simulink library "motor_lib"  (Simulink 7.8)
settings: Solver=ode45  StartTime=0.0  StopTime=10.0  RelTol=1e-3
libraries: powerlib x8
settings Model: Creator=re25624  LastModifiedBy=ma25949

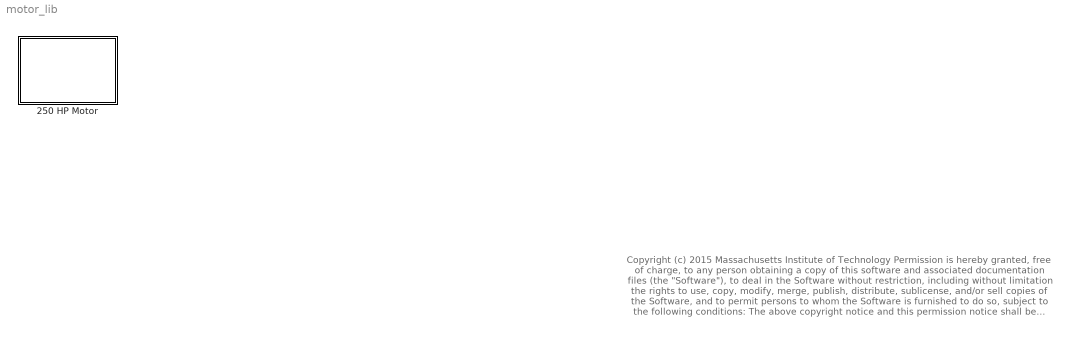
== system motor_lib ==
  note: Copyright (c) 2015 Massachusetts Institute of Technology
      | Permission is hereby granted, free of charge, to any person obtaining a copy of this software and associated documentation files (the "Software"), to deal in the Software without restriction, including without limitation the rights to use, copy, modify, merge, publish, distribute, sublicense, and/or sell copies of the Software, and to permit persons to whom the Software is furnished to do so, subject to the following conditions:
      |
      | The above copyright notice and this permission notice shall be included in all copies or substantial portions of the Software.
      |
      | THE SOFTWARE IS PROVIDED "AS IS", WITHOUT WARRANTY OF ANY KIND, EXPRESS OR IMPLIED, INCLUDING BUT NOT LIMITED TO THE WARRANTIES OF MERCHANTABILITY, FITNESS FOR A PARTICULAR PURPOSE AND NONINFRINGEMENT. IN NO EVENT SHALL THE AUTHORS OR COPYRIGHT HOLDERS BE LIABLE FOR ANY CLAIM,
      | DAMAGES OR OTHER LIABILITY, WHETHER IN AN ACTION OF CONTRACT, TORT OR OTHERWISE, ARISING FROM, OUT OF OR IN CONNECTION WITH THE SOFTWARE OR THE USE OR OTHER DEALINGS IN THE SOFTWARE.
  250 HP Motor : Subsystem  mask(SimPowersystems 250 HP custom motor){H=0.03}
      mask prompts: H "Inertia [Sec]"
      mask help:
      | This motor was built using parameters from the EPTM motor models.
      |
      | To keep this model stable, the inertia must be suffiently high. Otherwise, after the initial step the solution will be invalid and noisy. Also note that adding input filters appears to cause the solution to ring.
      |
      | When connecting this motor to an inductive load (such as a transformer), a capacitive load is necessary for the solvers to work properly.
      mask Display:
      | disp('250 HP\nmotor')
      | port_label('LConn', 1, 'A')
      | port_label('LConn', 2, 'B')
      | port_label('LConn', 3, 'C')

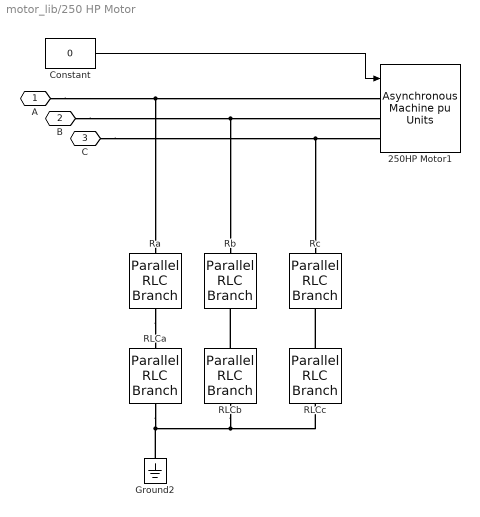
== system motor_lib/250 HP Motor ==
  250HP Motor1 : powerlib/Machines/Asynchronous Machine pu Units  PresetModel=No  MechanicalLoad=Torque Tm  ShowDetailedParameters=on  RotorType=Squirrel-cage  ReferenceFrame=Synchronous  NominalParameters=[187e3 460 60]  Stator=[0.0256294 0.0998644]  Rotor=[0.0100649 0.0998644]  Cage1=[0.01909 0.0397]  Cage2=[0.01909 0.0397]  Lm=3.47857  Mechanical=[H 0.005479 4]  PolePairs=4  InitialConditions="[ 1,0   0,0,0   0,0,0 ]"  Units=pu  LoadFlowParameters=0  SimulateSaturation=off  Saturation="[0.212,0.4201,0.8125,1.0979,1.4799,2.2457,3.2586,4.5763,6.4763 ;   0.5,0.7,0.9,1,1.1,1.2 ,1.3,1.4,1.5]"  TsPowergui=0  TsBlock=-1  IterativeModel=Forward Euler  Pmec=0
  Constant : Constant  Value=0
  Ground2 : powerlib/Elements/Ground  LConnTagsString=a
  RLCa : powerlib/Elements/Parallel RLC Branch  LConnTagsString=a  RConnTagsString=__new0  BranchType=RLC  Resistance=1e6  Inductance=inf  SetiL0=off  InitialCurrent=0  Capacitance=10e-6  Setx0=off  InitialVoltage=0  Measurements=None
  RLCb : powerlib/Elements/Parallel RLC Branch  LConnTagsString=a  RConnTagsString=__new0  BranchType=RLC  Resistance=1e6  Inductance=inf  SetiL0=off  InitialCurrent=0  Capacitance=10e-6  Setx0=off  InitialVoltage=0  Measurements=None
  "RLCc " : powerlib/Elements/Parallel RLC Branch  LConnTagsString=a  RConnTagsString=__new0  BranchType=RLC  Resistance=1e6  Inductance=inf  SetiL0=off  InitialCurrent=0  Capacitance=10e-6  Setx0=off  InitialVoltage=0  Measurements=None
  Ra : powerlib/Elements/Parallel RLC Branch  LConnTagsString=a  RConnTagsString=__new0  BranchType=R  Resistance=10e-3  Inductance=inf  SetiL0=off  InitialCurrent=0  Capacitance=0  Setx0=off  InitialVoltage=0  Measurements=None
  Rb : powerlib/Elements/Parallel RLC Branch  LConnTagsString=a  RConnTagsString=__new0  BranchType=R  Resistance=10e-3  Inductance=inf  SetiL0=off  InitialCurrent=0  Capacitance=0  Setx0=off  InitialVoltage=0  Measurements=None
  Rc : powerlib/Elements/Parallel RLC Branch  LConnTagsString=a  RConnTagsString=__new0  BranchType=R  Resistance=10e-3  Inductance=inf  SetiL0=off  InitialCurrent=0  Capacitance=0  Setx0=off  InitialVoltage=0  Measurements=None
  A : PMIOPort  Port=1  Side=Left
  B : PMIOPort  Port=2  Side=Left
  C : PMIOPort  Port=3  Side=Left
  wires:
  Constant/1 -> 250HP Motor1/1
  connections:
  C/RConn1 -- 250HP Motor1/LConn3 -- Rc/LConn1
  B/RConn1 -- 250HP Motor1/LConn2 -- Rb/LConn1
  A/RConn1 -- 250HP Motor1/LConn1 -- Ra/LConn1
  "RLCc "/RConn1 -- RLCb/RConn1 -- Ground2/LConn1 -- RLCa/RConn1
  RLCb/LConn1 -- Rb/RConn1
  Ra/RConn1 -- RLCa/LConn1
  "RLCc "/LConn1 -- Rc/RConn1
